simulink library "Controller_Wrapper"  (R2016b)
settings: Solver=VariableStepAuto  StartTime=0.0  StopTime=10.0  RelTol=1e-3
libraries: Controller_Wrapper x1
settings Model: Creator=UAVLAB  LastModifiedBy=rega0051

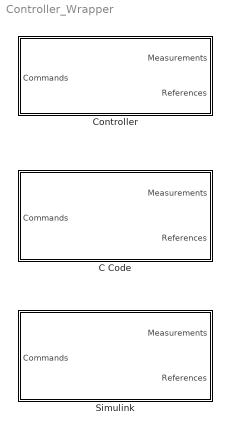
== system Controller_Wrapper ==
  C Code : Subsystem
  Controller : Subsystem  BlockChoice=C Code
      settings: TemplateBlock=self  MemberBlocks=C Code,Simulink
  Simulink : Subsystem

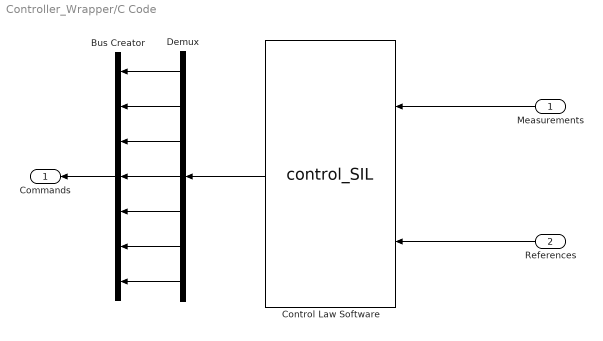
== system Controller_Wrapper/C Code ==
  Measurements : Inport  OutDataTypeStr=Bus: Sensors
  References : Inport  Port=2  OutDataTypeStr=Bus: Refs
  Bus Creator : BusCreator  Inputs=7  OutDataTypeStr=Bus: Commands
      settings: InheritFromInputs=off
  Control Law Software : S-Function  FunctionName=control_SIL  Parameters=SampleTime  SFunctionDeploymentMode=off  EnableBusSupport=off
  Demux : Demux  Outputs=7
  Commands : Outport  OutDataTypeStr=Bus: Commands
  wires:
  Measurements/1 -> Control Law Software/1
  References/1 -> Control Law Software/2
  Bus Creator/1 -> Commands/1
  Demux/7 -> Bus Creator/7
  Demux/6 -> Bus Creator/6
  Demux/5 -> Bus Creator/5
  Demux/4 -> Bus Creator/4
  Demux/3 -> Bus Creator/3
  Demux/2 -> Bus Creator/2
  Demux/1 -> Bus Creator/1
  Control Law Software/1 -> Demux/1

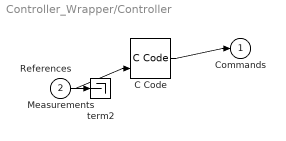
== system Controller_Wrapper/Controller ==
  Measurements : Inport
  References : Inport  Port=2
  C Code : Controller_Wrapper/C Code
  term2 : Terminator
  Commands : Outport
  wires:
  References/1 -> C Code/2
  C Code/1 -> Commands/1
  Measurements/1 -> term2/1

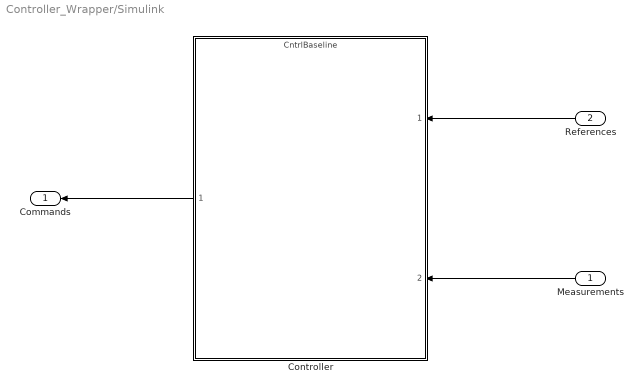
== system Controller_Wrapper/Simulink ==
  Measurements : Inport  OutDataTypeStr=Bus: Sensors
  References : Inport  Port=2  OutDataTypeStr=Bus: Refs
  Controller : ModelReference  ModelNameDialog=CntrlBaseline  SimulationMode=Normal  Variant=on  ModelReferenceVersion=1.58
  Commands : Outport  OutDataTypeStr=Bus: Commands
  wires:
  References/1 -> Controller/1
  Measurements/1 -> Controller/2
  Controller/1 -> Commands/1
